simulink model "L0304"  (R2015b)
settings: Solver=VariableStepAuto  SolverMode=SingleTasking  StartTime=0.0  StopTime=10.0  MaxStep=0.001  RelTol=1e-3
libraries: simulink x8
settings Model: Creator=Andrey  LastModifiedBy=mmf.shpakAV
settings DataIOCC: LimitDataPoints=off  ReturnWorkspaceOutputs=on
settings DebuggingCC: UnconnectedInputMsg=none  UnconnectedOutputMsg=none  UnconnectedLineMsg=none  AllowSymbolicDim=on  SFUnexpectedBacktrackingDiag=error  SFNoUnconditionalDefaultTransitionDiag=error
settings ModelReferenceCC: EnableRefExpFcnMdlSchedulingChecks=off  PropagateSignalLabelsOutOfModel=on
settings SFSimCC: SimUseLocalCustomCode=on
settings RTWCC: RTWUseLocalCustomCode=on
settings GRTTargetCC: TargetLangStandard=C99 (ISO)
settings ConfigComp: CovMetricSettings=dwe  CovSaveCumulativeToWorkspaceVar=off  CovSaveSingleToWorkspaceVar=off  CovModelRefEnable=Off  CovExternalEMLEnable=on

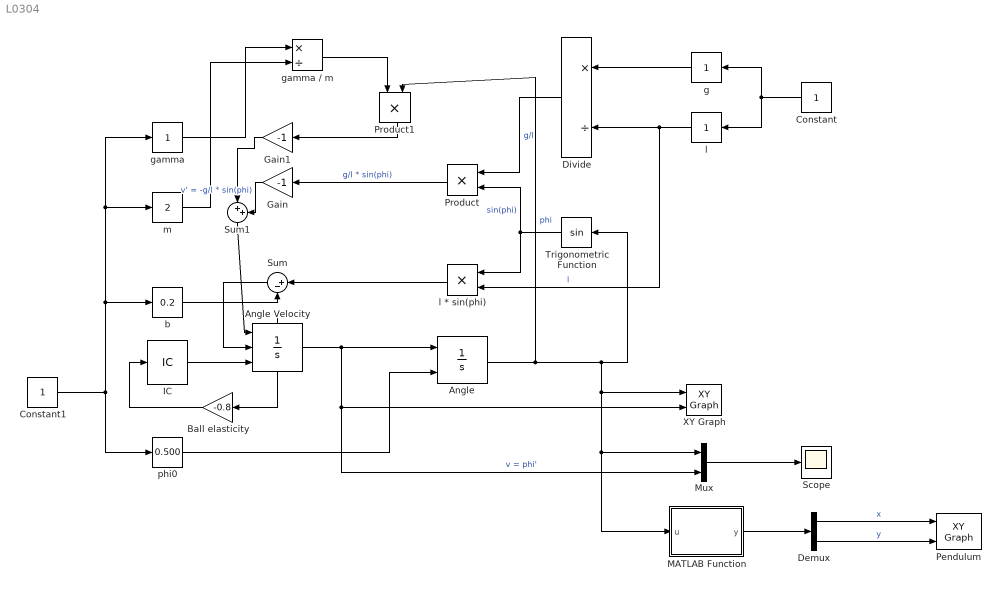
== system L0304 ==
  Angle : Integrator  InitialConditionSource=external
  Angle Velocity : Integrator  ExternalReset=falling  InitialConditionSource=external  ShowStatePort=on
  Ball elasticity : Gain  Gain=-0.8
  Constant : Constant
  Constant1 : Constant
  Demux : Demux  Outputs=2
  Divide : Product  Inputs=*/
  Gain : Gain  Gain=-1
  Gain1 : Gain  Gain=-1
  IC : InitialCondition  Value=0
  MATLAB Function : MATLAB Function  TreatAsAtomicUnit=on
  Mux : Mux  Inputs=2
  Pendulum : simulink/Sinks/XY Graph  xmin=-1  xmax=1  ymin=-1  ymax=1  st=-1
  Product : Product
  Product1 : Product
  Scope : Scope
  Sum : Sum  Inputs=|+-
  Sum1 : Sum  Inputs=|++
  Trigonometric Function : Trigonometry
  XY Graph : simulink/Sinks/XY Graph  xmin=-1  xmax=1  ymin=-1  ymax=1  st=-1
  b : simulink/Math Operations/Slider Gain  low=0  gain=0.2  high=2
  g : simulink/Math Operations/Slider Gain  low=0  gain=1  high=2
  gamma : simulink/Math Operations/Slider Gain  low=0  gain=1  high=2
  gamma / m : Product  Inputs=*/
  l : simulink/Math Operations/Slider Gain  low=0  gain=1  high=2
  l * sin(phi) : Product
  m : simulink/Math Operations/Slider Gain  low=0  gain=2  high=2
  phi0 : simulink/Math Operations/Slider Gain  low=0  gain=0.500  high=2
  wires:
  Angle Velocity/1 -> Angle/1, Mux/2, XY Graph/2  "v = phi'"
  Angle/1 -> Trigonometric Function/1, MATLAB Function/1(u), Mux/1, XY Graph/1, Product1/2  "phi"
  Constant/1 -> l/1, g/1
  g/1 -> Divide/1
  l/1 -> l * sin(phi)/2, Divide/2  "l"
  Trigonometric Function/1 -> l * sin(phi)/1, Product/2  "sin(phi)"
  Divide/1 -> Product/1  "g/l"
  Product/1 -> Gain/1  "g/l * sin(phi)"
  Mux/1 -> Scope/1
  IC/1 -> Angle Velocity/3
  phi0/1 -> Angle/2
  Constant1/1 -> phi0/1, gamma/1, m/1, b/1
  MATLAB Function/1(y) -> Demux/1
  Demux/1 -> Pendulum/1  "x"
  Demux/2 -> Pendulum/2  "y"
  l * sin(phi)/1 -> Sum/1
  b/1 -> Sum/2
  Sum/1 -> Angle Velocity/2
  Angle Velocity/State -> Ball elasticity/1
  Ball elasticity/1 -> IC/1
  gamma/1 -> gamma / m/1
  m/1 -> gamma / m/2
  gamma / m/1 -> Product1/1
  Product1/1 -> Gain1/1
  Gain1/1 -> Sum1/1
  Gain/1 -> Sum1/2  "v' = -g/l * sin(phi)"
  Sum1/1 -> Angle Velocity/1

== matlab function L0304/MATLAB Function ==
  data: u input; y output
function y  = fcn(u)
%#codegen

y = [sin(u),-cos(u)]';
